simulink model "platoon3"  (R2021a)
settings: Solver=VariableStepAuto  StartTime=0.0  StopTime=10.0  RelTol=1e-3
settings Model: Creator=shan  LastModifiedBy=shan
settings SolverCC: AlgebraicLoopSolver=TrustRegion
settings DebuggingCC: SFMachineParentedDataDiag=warning  UnderSpecifiedDimensionMsg=warning
settings ConfigComp: DVTestSuiteOptimization=Auto  DVDetectOutOfBounds=on

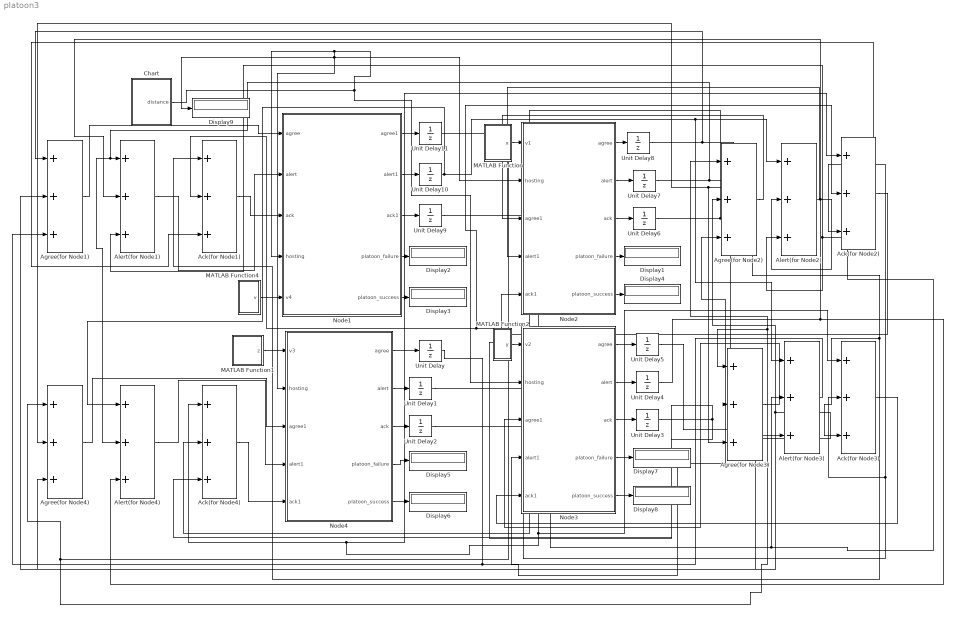
== system platoon3 ==
  Ack(for Node1) : Sum  Inputs=+++
  Ack(for Node2) : Sum  Inputs=+++
  Ack(for Node3) : Sum  Inputs=+++
  Ack(for Node4) : Sum  Inputs=+++
  Agree(for Node1) : Sum  Inputs=+++
  Agree(for Node2) : Sum  Inputs=+++
  Agree(for Node3) : Sum  Inputs=+++
  Agree(for Node4) : Sum  Inputs=+++
  Alert(for Node1) : Sum  Inputs=+++
  Alert(for Node2) : Sum  Inputs=+++
  Alert(for Node3) : Sum  Inputs=+++
  Alert(for Node4) : Sum  Inputs=+++
  Chart : Stateflow chart  TreatAsAtomicUnit=on
  Display{1..9} (9 alike) : Display
  MATLAB Function : MATLAB Function  TreatAsAtomicUnit=on
  MATLAB Function1 : MATLAB Function  TreatAsAtomicUnit=on
  MATLAB Function2 : MATLAB Function  TreatAsAtomicUnit=on
  MATLAB Function4 : MATLAB Function  TreatAsAtomicUnit=on
  Node1 : Stateflow chart  TreatAsAtomicUnit=on
      settings: PortSchema="{\"entries\":[{\"content\":{\"sides\":[{\"content\":{\"connectorIds\":[\"In1\",\"In2\",\"In3\",\"In4\",\"In5\"]},\"type\":\"ConnectorPlacement.EquallySpacedRectSide\",\"uuid\":\"734fbdd0-9501-4fb3-a80e-b93ab60da9cd\"},{\"content\":{\"connectorIds\":[\"Out3\",\"Out4\",\"Out5\",\"Out1\",\"Out2\"],\"side\":\"RIGHT\"},\"type\":\"ConnectorPlacement.EquallySpacedRectSide\",\"uuid\":\"5fc245a7-62da-4c1d-8651-4c21304ad71c\"},{\"content\":{\"connectorIds\":[],\"side\":\"TOP\"},\"type\":\"ConnectorPlacement.EquallySpacedRectSide\",\"uuid\":\"585259d6-d979-44e7-8a15-28144377417d\"},{\"content\":{\"connectorIds\":[],\"side\":\"HIDDEN\"},\"type\":\"ConnectorPlacement.EquallySpacedRectSide\",\"uuid\":\"c5d86299-f8c2-46f3-82a7-6a0d37049aa8\"}]},\"type\":\"ConnectorPlacement.EquallySpacedConnector\",\"uuid\":\"8535649b-8615-4473-b4f1-0f1d9df57b0a\"}],\"packageUris\":[\"http://schema.mathworks.com/mf0/Connector/R2020b\"],\"version\":\"1.0\"}"
  Node2 : Stateflow chart  TreatAsAtomicUnit=on
  Node3 : Stateflow chart  TreatAsAtomicUnit=on
  Node4 : Stateflow chart  TreatAsAtomicUnit=on
  Unit Delay{,1..11} (12 alike) : UnitDelay  SampleTime=-1  HasFrameUpgradeWarning=on
  wires:
  Node1/1(platoon_failure) -> Display2/1
  Node1/2(platoon_success) -> Display3/1
  Node2/1(agree) -> Unit Delay8/1
  Node3/1(agree) -> Unit Delay5/1
  Node4/1(agree) -> Unit Delay/1
  Agree(for Node1)/1 -> Node1/1(agree)
  MATLAB Function/1(x) -> Node2/1(v1)
  MATLAB Function1/1(z) -> Node4/1(v3)
  MATLAB Function2/1(y) -> Node3/1(v2)
  Node3/2(alert) -> Unit Delay4/1
  Node4/3(ack) -> Unit Delay2/1
  Node3/3(ack) -> Unit Delay3/1
  Node4/2(alert) -> Unit Delay1/1
  Node2/3(ack) -> Unit Delay6/1
  Node2/2(alert) -> Unit Delay7/1
  Alert(for Node1)/1 -> Node1/2(alert)
  Ack(for Node1)/1 -> Node1/3(ack)
  Node2/4(platoon_failure) -> Display1/1
  Node2/5(platoon_success) -> Display4/1
  Node4/4(platoon_failure) -> Display5/1
  Node4/5(platoon_success) -> Display6/1
  Node3/4(platoon_failure) -> Display7/1
  Node3/5(platoon_success) -> Display8/1
  Node1/3(agree1) -> Unit Delay11/1
  Node1/4(alert1) -> Unit Delay10/1
  Node1/5(ack1) -> Unit Delay9/1
  Agree(for Node2)/1 -> Node2/3(agree1)
  Alert(for Node2)/1 -> Node2/4(alert1)
  Ack(for Node2)/1 -> Node2/5(ack1)
  Ack(for Node3)/1 -> Node3/5(ack1)
  Alert(for Node3)/1 -> Node3/4(alert1)
  Agree(for Node3)/1 -> Node3/3(agree1)
  Ack(for Node4)/1 -> Node4/5(ack1)
  Alert(for Node4)/1 -> Node4/4(alert1)
  Agree(for Node4)/1 -> Node4/3(agree1)
  MATLAB Function4/1(v) -> Node1/5(v4)
  Unit Delay/1 -> Agree(for Node3)/2, Agree(for Node2)/3, Agree(for Node1)/3
  Unit Delay1/1 -> Alert(for Node1)/3, Alert(for Node2)/3, Alert(for Node3)/2
  Unit Delay2/1 -> Ack(for Node1)/3, Ack(for Node2)/3, Ack(for Node3)/2
  Unit Delay5/1 -> Agree(for Node1)/2, Agree(for Node2)/2, Agree(for Node4)/3
  Unit Delay4/1 -> Alert(for Node4)/3, Alert(for Node1)/2, Alert(for Node2)/2
  Unit Delay3/1 -> Ack(for Node4)/3, Ack(for Node1)/2, Ack(for Node2)/2
  Unit Delay8/1 -> Agree(for Node4)/2, Agree(for Node3)/3, Agree(for Node1)/1
  Unit Delay7/1 -> Alert(for Node4)/2, Alert(for Node1)/1, Alert(for Node3)/3
  Unit Delay6/1 -> Ack(for Node1)/1, Ack(for Node3)/3, Ack(for Node4)/2
  Unit Delay11/1 -> Agree(for Node4)/1, Agree(for Node2)/1, Agree(for Node3)/1
  Unit Delay10/1 -> Alert(for Node3)/1, Alert(for Node2)/1, Alert(for Node4)/1
  Unit Delay9/1 -> Ack(for Node4)/1, Ack(for Node2)/1, Ack(for Node3)/1
  Chart/1(distance) -> Node3/2(hosting), Node1/4(hosting), Node2/2(hosting), Display9/1, Node4/2(hosting)

== stateflow chart platoon3/Node3 ==
  state Agend
    state Inactive
      state Ready
        entry:
        agree = 1;
      state Init
        entry:
        dead = false;
      state Wait
      (default) -> Agend.Inactive.Init
      Agend.Inactive.Wait -> Agend.Inactive.Ready : [dead == false]
      Agend.Inactive.Init -> Agend.Inactive.Wait
    state Active
      state Platoon
        entry:
        platoon_function();
      state platoon_function [function]
        (default) -> (junction 191)
        (junction 191) -> (junction 192) [order 1] : [v2 > 50]
        (junction 191) -> (junction 193) [order 2] : {alert = 1;}
        (junction 192) -> (junction 194) : {ack = 1;}
        (junction 194) -> (junction 193)
        (junction 193) -> (junction 195)
    (default) -> Agend.Inactive
    Agend.Inactive.Ready -> Platoon
  state Host
    state Init
      entry:
      platoon_success=0;
      platoon_failure=0;
    state Commit
      entry:
    state PTC
    state Success
      entry:
      platoon_failure = alert1;
      platoon_success = ack1;
    state Fail
      entry:
      platoon_failure = alert1;
      platoon_success = ack1;
    (default) -> Host.Init
    Host.Init -> Host.PTC
    Host.PTC -> Host.Commit : [agree1 >= 2]
    Host.Commit -> Host.Success [order 1] : [ack1 >= 2]
    Host.Commit -> Host.Fail [order 2] : [alert1 >= 2]
  state Agend1 [commented out]
    state Inactive [commented out]
      state Ready [commented out]
        entry:
        agree = 1;
      state Init [commented out]
        entry:
        dead = false;
      state Ok [commented out]
        entry:
        alert = 0;
        ack = 1;
        jackH=jackH + 1;
        v1
      state Wait [commented out]
      state Zero [commented out]
        entry:
        rH_jack = 0;
        jackH = 0;
        dead = false;
        alert = 0;
      state Fault [commented out]
        entry:
        alert=1;
        ack=0;
        dead=true;
      state Init1 [commented out]
        entry:
        rH_jack = 0;
        jackH = 0;
        dead = false;
      (default) -> Agend1.Inactive.Init [commented out]
      Agend1.Inactive.Wait -> Agend1.Inactive.Ready [commented out] : [prepare == 1 && dead == false]
      Agend1.Inactive.Init -> Agend1.Inactive.Wait [commented out]
      Ok -> Agend1.Inactive.Wait [commented out] : [reset==0]
      Zero -> Agend1.Inactive.Wait [commented out]
      Ok -> Zero [commented out]
      Fault -> Zero [commented out] : [reset==1]
    state Active [commented out]
      state Lift [commented out]
        entry:
        lift_function();
      state lift_function [function] [commented out]
        (default) -> (junction 277) [commented out]
        (junction 277) -> (junction 278) [commented out] : [v2 > 50]
        (junction 277) -> (junction 279) [commented out] : {alert = 1;}
        (junction 278) -> (junction 280) [commented out] : {ack = 1;}
        (junction 280) -> (junction 279) [commented out]
        (junction 279) -> (junction 281) [commented out]
    (default) -> Agend1.Inactive [commented out]
    Agend1.Inactive.Ready -> Lift [commented out]
    Lift -> Fault [commented out]
    Lift -> Ok [commented out] : [rH_jack == jackH +1]
  state Host1 [commented out]
    state Init [commented out]
      entry:
      platoon_success=0;
      platoon_failure=0;
    state Commit [commented out]
      entry:
    state PTC [commented out]
      entry: prepare = 1;
    state End_lift [commented out]
      entry:
      num_failure = 0;
      total_height = total_height +1;
    state Go_to_zero [commented out]
      entry:
      num_failure = num_failure + 1;
      reset = 1;
    state Commit1 [commented out]
      entry:
      commit = 0;
    state Success [commented out]
      entry:
      platoon_failure = alert1;
      platoon_success = ack1;
    state Fail [commented out]
      entry:
      platoon_failure = alert1;
      platoon_success = ack1;
    (default) -> Host1.Init [commented out]
    End_lift -> Host1.PTC [commented out] : [total_height<15]
    Host1.Init -> Host1.PTC [commented out]
    Host1.PTC -> Host1.Commit [commented out] : [agree1 >= 2]
    Host1.Commit -> End_lift [commented out] : [alert < 1 && alert + ack == 4]
    Host1.Commit -> Host1.Success [commented out] : [ack1 >= 2]
    Host1.Commit -> Go_to_zero [commented out] : [alert >= 3 && alert + ack == 4]
    Host1.Commit -> Host1.Fail [commented out] : [alert1 >= 2]
    Host1.PTC -> Commit1 [commented out] : [agree < 2]
    Go_to_zero -> Host1.PTC [commented out]
    End_lift -> Host1.Success [commented out]
    Go_to_zero -> Host1.Fail [commented out] : [num_failure == 3]
  (default) -> Host
  Agend -> Host : [hosting >= 50 && hosting <= 74]
  Host -> Agend : [~(hosting >= 50 && hosting <= 74)]
  (default) -> Host1 [commented out]
  Agend1 -> Host1 [commented out] : [hosting >= 50 && hosting <= 74]
  Host1 -> Agend1 [commented out] : [~(hosting >= 50 && hosting <= 74)]
  data: agree output; dead local; v2 input; alert output; ack output; hosting input; agree1 input; alert1 input; ack1 input; platoon_failure output; platoon_success output

== stateflow chart platoon3/Node4 ==
  state Host
    state Init
      entry:
      platoon_success=0;
      platoon_failure=0;
    state Commit
    state PTC
    state Success
      entry:
      platoon_failure = alert1;
      platoon_success = ack1;
    state Fail
      entry:
      platoon_failure = alert1;
      platoon_success = ack1;
    (default) -> Host.Init
    Host.Init -> Host.PTC
    Host.PTC -> Host.Commit : [agree1 >= 2]
    Host.Commit -> Host.Fail [order 2] : [alert1 >= 2]
    Host.Commit -> Host.Success [order 1] : [ack1 >= 2]
  state Agend
    state Inactive
      state Ready
        entry:
        agree = 1;
      state Init
        entry:
        dead = false;
      state Wait
      (default) -> Agend.Inactive.Init
      Agend.Inactive.Wait -> Agend.Inactive.Ready : [dead == false]
      Agend.Inactive.Init -> Agend.Inactive.Wait
    state Active
      state Platoon
        entry:
        platoon_function();
      state platoon_function [function]
        (default) -> (junction 157)
        (junction 157) -> (junction 158) [order 1] : [v3 > 50]
        (junction 157) -> (junction 159) [order 2] : {alert = 1;}
        (junction 158) -> (junction 160) : {ack = 1;}
        (junction 160) -> (junction 159)
        (junction 159) -> (junction 161)
    (default) -> Agend.Inactive
    Agend.Inactive.Ready -> Platoon
  state Host1 [commented out]
    state Init [commented out]
      entry:
      platoon_success=0;
      platoon_failure=0;
    state Commit [commented out]
    state PTC [commented out]
      entry: prepare = 1;
    state End_lift [commented out]
      entry:
      num_failure = 0;
      total_height = total_height +1;
    state Go_to_zero [commented out]
      entry:
      num_failure = num_failure + 1;
      reset = 1;
    state Commit1 [commented out]
      entry:
      commit = 0;
    state Success [commented out]
      entry:
      platoon_failure = alert1;
      platoon_success = ack1;
    state Fail [commented out]
      entry:
      platoon_failure = alert1;
      platoon_success = ack1;
    (default) -> Host1.Init [commented out]
    End_lift -> Host1.PTC [commented out] : [total_height<15]
    Host1.Init -> Host1.PTC [commented out]
    Host1.PTC -> Host1.Commit [commented out] : [agree1 >= 2]
    Host1.Commit -> End_lift [commented out] : [alert < 1 && alert + ack == 4]
    Host1.Commit -> Go_to_zero [commented out] : [alert >= 3 && alert + ack == 4]
    Host1.Commit -> Host1.Fail [commented out] : [alert1 >= 2]
    Host1.Commit -> Host1.Success [commented out] : [ack1 >= 2]
    Host1.PTC -> Commit1 [commented out] : [agree < 2]
    Go_to_zero -> Host1.PTC [commented out]
    End_lift -> Host1.Success [commented out]
    Go_to_zero -> Host1.Fail [commented out] : [num_failure == 3]
  state Agend1 [commented out]
    state Inactive [commented out]
      state Ready [commented out]
        entry:
        agree = 1;
      state Init [commented out]
        entry:
        dead = false;
      state Ok [commented out]
        entry:
        alert = 0;
        ack = 1;
        jackH=jackH + 1;
        v1
      state Wait [commented out]
      state Zero [commented out]
        entry:
        rH_jack = 0;
        jackH = 0;
        dead = false;
        alert = 0;
      state Fault [commented out]
        entry:
        alert=1;
        ack=0;
        dead=true;
      state Init1 [commented out]
        entry:
        rH_jack = 0;
        jackH = 0;
        dead = false;
      (default) -> Agend1.Inactive.Init [commented out]
      Agend1.Inactive.Wait -> Agend1.Inactive.Ready [commented out] : [prepare == 1 && dead == false]
      Agend1.Inactive.Init -> Agend1.Inactive.Wait [commented out]
      Ok -> Agend1.Inactive.Wait [commented out] : [reset==0]
      Zero -> Agend1.Inactive.Wait [commented out]
      Ok -> Zero [commented out]
      Fault -> Zero [commented out] : [reset==1]
    state Active [commented out]
      state Lift [commented out]
        entry:
        lift_function();
      state lift_function [function] [commented out]
        (default) -> (junction 246) [commented out]
        (junction 246) -> (junction 247) [commented out] : [v3 > 50]
        (junction 246) -> (junction 248) [commented out] : {alert = 1;}
        (junction 247) -> (junction 249) [commented out] : {ack = 1;}
        (junction 249) -> (junction 248) [commented out]
        (junction 248) -> (junction 250) [commented out]
    (default) -> Agend1.Inactive [commented out]
    Agend1.Inactive.Ready -> Lift [commented out]
    Lift -> Fault [commented out]
    Lift -> Ok [commented out] : [rH_jack == jackH +1]
  (default) -> Agend
  Agend -> Host : [hosting >= 75]
  Host -> Agend : [~(hosting >= 75)]
  (default) -> Agend1 [commented out]
  Agend1 -> Host1 [commented out] : [hosting >= 75]
  Host1 -> Agend1 [commented out] : [~(hosting >= 75)]
  data: agree output; dead local; v3 input; alert output; ack output; hosting input; agree1 input; alert1 input; ack1 input; platoon_failure output; platoon_success output

== stateflow chart platoon3/Node1 ==
  state agend
    state Inactive
      state Ready
        entry:
        agree1 = 1;
      state Init
        entry:
        dead = false;
      state Wait
      (default) -> agend.Inactive.Init
      agend.Inactive.Wait -> agend.Inactive.Ready : [dead == false]
      agend.Inactive.Init -> agend.Inactive.Wait
    state Active
      state Platoon
        entry:
        platoon_function();
      state platoon_function [function]
        (default) -> (junction 136)
        (junction 136) -> (junction 137) [order 1] : [v4 > 50]
        (junction 136) -> (junction 138) [order 2] : {alert1 = 1;}
        (junction 137) -> (junction 120) : {ack1 = 1;}
        (junction 120) -> (junction 138)
        (junction 138) -> (junction 121)
    (default) -> agend.Inactive
    agend.Inactive.Ready -> Platoon
  state Host
    state Init
      entry:
      platoon_success=0;
      platoon_failure=0;
    state Commit
    state PTC
    state Success
      entry:
      platoon_success = ack;
      platoon_failure = alert;
    state Fail
      entry:
      platoon_success = ack;
      platoon_failure = alert;
    (default) -> Host.Init
    Host.Init -> Host.PTC
    Host.PTC -> Host.Commit : [agree >= 2]
    Host.Commit -> Host.Fail [order 2] : [alert >= 2]
    Host.Commit -> Host.Success [order 1] : [ack >= 2]
  state agend1 [commented out]
    state Inactive [commented out]
      state Ready [commented out]
        entry:
        agree1 = 1;
      state Init [commented out]
        entry:
        dead = false;
      state Ok [commented out]
        entry:
        alert = 0;
        ack = 1;
        jackH=jackH + 1;
        v1
      state Wait [commented out]
      state Zero [commented out]
        entry:
        rH_jack = 0;
        jackH = 0;
        dead = false;
        alert = 0;
      state Fault [commented out]
        entry:
        alert=1;
        ack=0;
        dead=true;
      state Init1 [commented out]
        entry:
        rH_jack = 0;
        jackH = 0;
        dead = false;
      (default) -> agend1.Inactive.Init [commented out]
      agend1.Inactive.Wait -> agend1.Inactive.Ready [commented out] : [prepare == 1 && dead == false]
      agend1.Inactive.Init -> agend1.Inactive.Wait [commented out]
      Ok -> agend1.Inactive.Wait [commented out] : [reset==0]
      Zero -> agend1.Inactive.Wait [commented out]
      Ok -> Zero [commented out]
      Fault -> Zero [commented out] : [reset==1]
    state Active [commented out]
      state Lift [commented out]
        entry:
        lift_function();
      state lift_function [function] [commented out]
        (default) -> (junction 178) [commented out]
        (junction 178) -> (junction 179) [commented out] : [v4 > 50]
        (junction 178) -> (junction 180) [commented out] : {alert1 = 1;}
        (junction 179) -> (junction 181) [commented out] : {ack1 = 1;}
        (junction 181) -> (junction 180) [commented out]
        (junction 180) -> (junction 182) [commented out]
    (default) -> agend1.Inactive [commented out]
    agend1.Inactive.Ready -> Lift [commented out]
    Lift -> Fault [commented out]
    Lift -> Ok [commented out] : [rH_jack == jackH +1]
  state Host1 [commented out]
    state Init [commented out]
      entry:
      platoon_success=0;
      platoon_failure=0;
    state Commit [commented out]
    state PTC [commented out]
      entry: prepare = 1;
    state End_lift [commented out]
      entry:
      num_failure = 0;
      total_height = total_height +1;
    state Go_to_zero [commented out]
      entry:
      num_failure = num_failure + 1;
      reset = 1;
    state Commit1 [commented out]
      entry:
      commit = 0;
    state Success [commented out]
      entry:
      platoon_success = ack;
      platoon_failure = alert;
    state Fail [commented out]
      entry:
      platoon_success = ack;
      platoon_failure = alert;
    (default) -> Host1.Init [commented out]
    End_lift -> Host1.PTC [commented out] : [total_height<15]
    Host1.Init -> Host1.PTC [commented out]
    Host1.PTC -> Host1.Commit [commented out] : [agree >= 2]
    Host1.Commit -> End_lift [commented out] : [alert < 1 && alert + ack == 4]
    Host1.Commit -> Go_to_zero [commented out] : [alert >= 3 && alert + ack == 4]
    Host1.Commit -> Host1.Fail [commented out] : [alert >= 2]
    Host1.Commit -> Host1.Success [commented out] : [ack >= 2]
    Host1.PTC -> Commit1 [commented out] : [agree < 2]
    Go_to_zero -> Host1.PTC [commented out]
    End_lift -> Host1.Success [commented out]
    Go_to_zero -> Host1.Fail [commented out] : [num_failure == 3]
  (default) -> Host
  agend -> Host : [hosting > 0 && hosting < 24]
  Host -> agend : [~(hosting > 0 && hosting < 24)]
  (default) -> Host1 [commented out]
  agend1 -> Host1 [commented out] : [hosting > 0 && hosting < 24]
  Host1 -> agend1 [commented out] : [~(hosting > 0 && hosting < 24)]
  data: agree input; platoon_failure output; platoon_success output; alert input; ack input; hosting input; agree1 output; alert1 output; ack1 output; dead local; v4 input

== stateflow chart platoon3/Node2 ==
  state Host
    state Init
      entry:
      platoon_success=0;
      platoon_failure=0;
    state Commit
    state PTC
    state Success
      entry:
      platoon_failure = alert1;
      platoon_success = ack1;
    state Fail
      entry:
      platoon_failure = alert1;
      platoon_success = ack1;
    (default) -> Host.Init
    Host.Init -> Host.PTC
    Host.PTC -> Host.Commit : [agree1 >= 2]
    Host.Commit -> Host.Success [order 1] : [ack1 >= 2]
    Host.Commit -> Host.Fail [order 2] : [alert1 >= 2]
  state Agend
    state Inactive
      state Ready
        entry:
        agree = 1;
      state Init
        entry:
        dead = false;
      state Wait
      (default) -> Agend.Inactive.Init
      Agend.Inactive.Wait -> Agend.Inactive.Ready : [dead == false]
      Agend.Inactive.Init -> Agend.Inactive.Wait
    state Active
      state Platoon
        entry:
        platoon_function();
      state platoon_function [function]
        (default) -> (junction 111)
        (junction 111) -> (junction 112) [order 1] : [v1 > 50]
        (junction 111) -> (junction 113) [order 2] : {alert = 1;}
        (junction 112) -> (junction 114) : {ack = 1;}
        (junction 114) -> (junction 113)
        (junction 113) -> (junction 115)
    (default) -> Agend.Inactive
    Agend.Inactive.Ready -> Platoon
  state Host1 [commented out]
    state Init [commented out]
      entry:
      platoon_success=0;
      platoon_failure=0;
    state Commit [commented out]
    state PTC [commented out]
      entry: prepare = 1;
    state End_lift [commented out]
      entry:
      num_failure = 0;
      total_height = total_height +1;
    state Go_to_zero [commented out]
      entry:
      num_failure = num_failure + 1;
      reset = 1;
    state Commit1 [commented out]
      entry:
      commit = 0;
    state Success [commented out]
      entry:
      platoon_failure = alert1;
      platoon_success = ack1;
    state Fail [commented out]
      entry:
      platoon_failure = alert1;
      platoon_success = ack1;
    (default) -> Host1.Init [commented out]
    End_lift -> Host1.PTC [commented out] : [total_height<15]
    Host1.Init -> Host1.PTC [commented out]
    Host1.PTC -> Host1.Commit [commented out] : [agree1 >= 2]
    Host1.Commit -> End_lift [commented out] : [alert < 1 && alert + ack == 4]
    Host1.Commit -> Host1.Success [commented out] : [ack1 >= 2]
    Host1.Commit -> Go_to_zero [commented out] : [alert >= 3 && alert + ack == 4]
    Host1.Commit -> Host1.Fail [commented out] : [alert1 >= 2]
    Host1.PTC -> Commit1 [commented out] : [agree < 2]
    Go_to_zero -> Host1.PTC [commented out]
    End_lift -> Host1.Success [commented out]
    Go_to_zero -> Host1.Fail [commented out] : [num_failure == 3]
  state Agend1 [commented out]
    state Inactive [commented out]
      state Ready [commented out]
        entry:
        agree = 1;
      state Init [commented out]
        entry:
        dead = false;
      state Ok [commented out]
        entry:
        alert = 0;
        ack = 1;
        jackH=jackH + 1;
        v1
      state Wait [commented out]
      state Zero [commented out]
        entry:
        rH_jack = 0;
        jackH = 0;
        dead = false;
        alert = 0;
      state Fault [commented out]
        entry:
        alert=1;
        ack=0;
        dead=true;
      state Init1 [commented out]
        entry:
        rH_jack = 0;
        jackH = 0;
        dead = false;
      (default) -> Agend1.Inactive.Init [commented out]
      Agend1.Inactive.Wait -> Agend1.Inactive.Ready [commented out] : [prepare == 1 && dead == false]
      Agend1.Inactive.Init -> Agend1.Inactive.Wait [commented out]
      Ok -> Agend1.Inactive.Wait [commented out] : [reset==0]
      Zero -> Agend1.Inactive.Wait [commented out]
      Ok -> Zero [commented out]
      Fault -> Zero [commented out] : [reset==1]
    state Active [commented out]
      state Lift [commented out]
        entry:
        lift_function();
      state lift_function [function] [commented out]
        (default) -> (junction 220) [commented out]
        (junction 220) -> (junction 221) [commented out] : [v1 > 50]
        (junction 220) -> (junction 222) [commented out] : {alert = 1;}
        (junction 221) -> (junction 223) [commented out] : {ack = 1;}
        (junction 223) -> (junction 222) [commented out]
        (junction 222) -> (junction 224) [commented out]
    (default) -> Agend1.Inactive [commented out]
    Agend1.Inactive.Ready -> Lift [commented out]
    Lift -> Fault [commented out]
    Lift -> Ok [commented out] : [rH_jack == jackH +1]
  (default) -> Host
  Agend -> Host : [hosting >= 25 && hosting <= 49]
  Host -> Agend : [~(hosting >= 25 && hosting <= 49)]
  (default) -> Host1 [commented out]
  Agend1 -> Host1 [commented out] : [hosting >= 25 && hosting <= 49]
  Host1 -> Agend1 [commented out] : [~(hosting >= 25 && hosting <= 49)]
  data: agree output; dead local; v1 input; alert output; ack output; hosting input; platoon_failure output; platoon_success output; agree1 input; alert1 input; ack1 input

== matlab function platoon3/MATLAB Function ==
  data: x output

function x = v1()

% a = 30;
% b= 100;
% 
% x = round((a + (b-a) .* rand(1,1)));
% 
% 
%  end
coder.extrinsic('rand','rng');
x = 0;

persistent atTime0
if isempty(atTime0)
    rng('shuffle');
    atTime0 = false;
end

x = round(rand * 100);

== matlab function platoon3/MATLAB Function1 ==
  data: z output
function z = v3()

% a = 25;
% b= 100;
% 
% z = round((a + (b-a) .* rand(1,1)));
% 
% end

coder.extrinsic('rand','rng');
z = 0;

persistent atTime0
if isempty(atTime0)
    rng('shuffle');
    atTime0 = false;
end

z = round(rand * 100);

== matlab function platoon3/MATLAB Function2 ==
  data: y output
function y = v2()

coder.extrinsic('rand','rng');
y = 0;

persistent atTime0
if isempty(atTime0)
    rng('shuffle');
    atTime0 = false;
end

y = round(rand * 100);

== matlab function platoon3/MATLAB Function4 ==
  data: v output
function v = v4()

coder.extrinsic('rand','rng');
v = 0;

persistent atTime0
if isempty(atTime0)
    rng('shuffle');
    atTime0 = false;
end

v = round(rand * 100);

== stateflow chart platoon3/Chart ==
  state Hosting_output
    entry:
    v9();
    distance = v9;
    state selct_host_name(out) [function] [commented out]
      (default) -> (junction 64) [commented out] : % Select Host Name
      (junction 64) -> (junction 65) [commented out] : [out > 0 && out < 24]
      (junction 64) -> (junction 66) [commented out]
      (junction 65) -> (junction 73) [commented out] : {Host = 1;}
      (junction 66) -> (junction 67) [commented out] : [out >= 25 && out <= 49]
      (junction 66) -> (junction 68) [commented out]
      (junction 67) -> (junction 72) [commented out] : {Host = 2;}
      (junction 68) -> (junction 69) [commented out] : [out >= 50 && out <= 74]
      (junction 68) -> (junction 70) [commented out] : {Host = 4;}
      (junction 69) -> (junction 71) [commented out] : {Host = 3;}
      (junction 71) -> (junction 70) [commented out]
      (junction 72) -> (junction 71) [commented out]
      (junction 73) -> (junction 72) [commented out]
      (junction 70) -> (junction 74) [commented out]
  (default) -> Hosting_output
  data: out function_input; x function_output; distance output
  function x = v9:
    | function x = v9()
    | 
    | % a = 30;
    | % b= 100;
    | % 
    | % x = round((a + (b-a) .* rand(1,1)));
    | % 
    | % 
    | %  end
    | coder.extrinsic('rand','rng');
    | x = 0;
    | 
    | persistent atTime0
    | if isempty(atTime0)
    |     rng('shuffle');
    |     atTime0 = false;
    | end
    | 
    | x = round(rand * 100);
